simulink model "A21_S7905713_S8999827"  (R2025b)
settings: Solver=VariableStepAuto  StartTime=0.0  StopTime=10.0  RelTol=1e-3
undefined symbols (not defined in the file): X, Y, Z
libraries: nesl_utility x31, sm_lib x27, robotcorelib x1, simulink x1
settings Model: Creator=lucaa  LastModifiedBy=lucaa

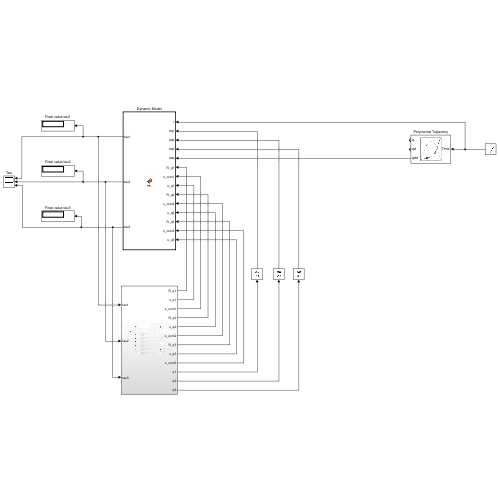
[thumbnail: Simulink's stored preview of the top-level diagram]
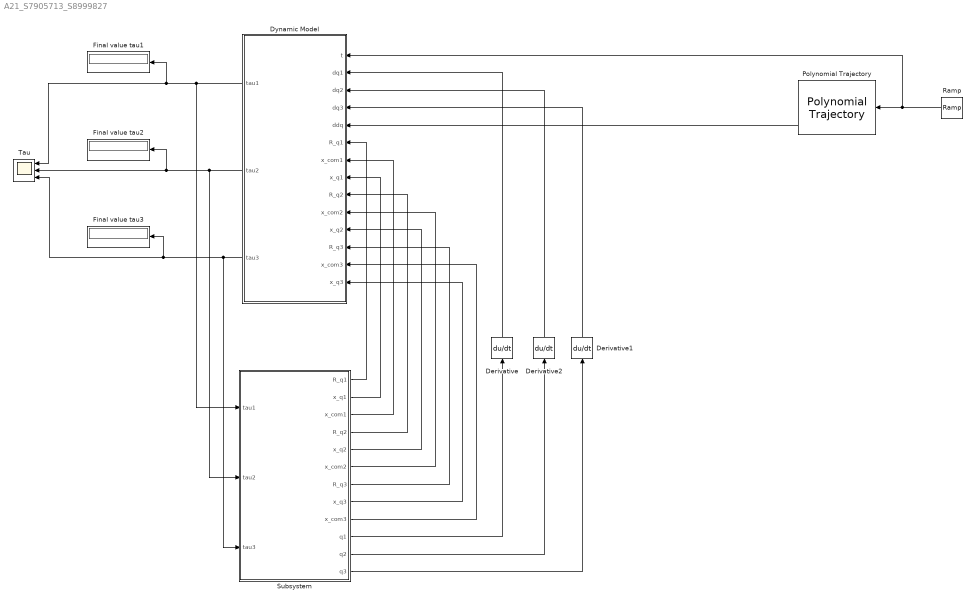
== system A21_S7905713_S8999827 ==
  Derivative : Derivative
  Derivative1 : Derivative
  Derivative2 : Derivative
  Dynamic Model : MATLAB Function  TreatAsAtomicUnit=on
  Final value tau1 : Display
  Final value tau2 : Display
  Final value tau3 : Display
  Polynomial Trajectory : robotcorelib/Polynomial Trajectory  WaypointSource=Internal  Waypoints=[pi/9,pi/3;pi/6,-(pi/180)*15;-(pi/18),(pi/9)*2]  TimePoints=[0,10]  TimeInterval=[ 1, 4 ]  Method=Cubic Polynomial  ParameterSource=Internal  VelocityBoundaryCondition=zeros( 3,2 )  AccelerationBoundaryCondition=zeros( 2, 5 )  SimulateUsing=Interpreted execution
  Ramp : simulink/Sources/Ramp  slope=1  start=0  InitialOutput=0
  Subsystem : Subsystem
  Tau : Scope  NumInputPorts=3
      settings: ActiveDisplayYMinimum=-52.940728526293412  ActiveDisplayYMaximum=68.833359173627684
  wires:
  Subsystem/6(x_com2) -> Dynamic Model/10(x_com2)
  Subsystem/1(R_q1) -> Dynamic Model/6(R_q1)
  Subsystem/4(R_q2) -> Dynamic Model/9(R_q2)
  Subsystem/3(x_com1) -> Dynamic Model/7(x_com1)
  Subsystem/5(x_q2) -> Dynamic Model/11(x_q2)
  Dynamic Model/1(tau1) -> Tau/1, Final value tau1/1, Subsystem/1(tau1)
  Subsystem/2(x_q1) -> Dynamic Model/8(x_q1)
  Dynamic Model/2(tau2) -> Tau/2, Final value tau2/1, Subsystem/2(tau2)
  Polynomial Trajectory/3 -> Dynamic Model/5(ddq)
  Subsystem/7(R_q3) -> Dynamic Model/12(R_q3)
  Subsystem/8(x_q3) -> Dynamic Model/14(x_q3)
  Subsystem/9(x_com3) -> Dynamic Model/13(x_com3)
  Dynamic Model/3(tau3) -> Final value tau3/1, Tau/3, Subsystem/3(tau3)
  Ramp/1 -> Polynomial Trajectory/1, Dynamic Model/1(t)
  Subsystem/10(q1) -> Derivative/1
  Derivative/1 -> Dynamic Model/2(dq1)
  Subsystem/11(q2) -> Derivative2/1
  Subsystem/12(q3) -> Derivative1/1
  Derivative2/1 -> Dynamic Model/3(dq2)
  Derivative1/1 -> Dynamic Model/4(dq3)

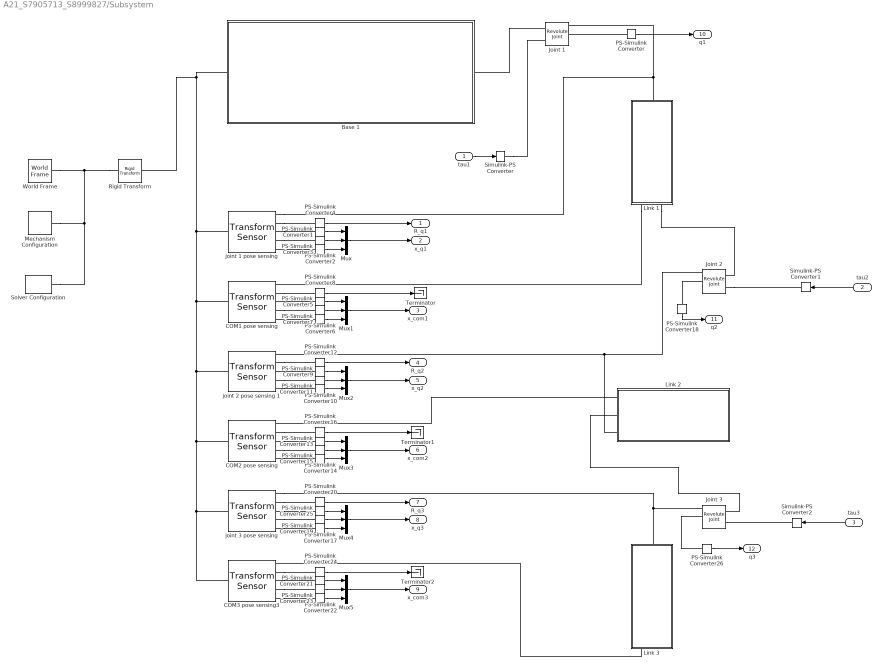
== system A21_S7905713_S8999827/Subsystem ==
  tau1 : Inport
  tau2 : Inport  Port=2
  tau3 : Inport  Port=3
  " Joint 1" : sm_lib/Joints/Revolute Joint  JointMode=Normal  CompositeWrenchDir=FollowerOnBase  CompositeWrenchFrame=BaseFrame  SenseConstraintForce=off  SenseConstraintTorque=off  SenseTotalForce=off  SenseTotalTorque=off  PositionTargetSpecify=on  PositionTargetPriority=High  PositionTargetValue=20  PositionTargetValueUnits=deg  VelocityTargetSpecify=off  VelocityTargetPriority=High  VelocityTargetValue=0  VelocityTargetValueUnits=deg/s  EquilibriumPosition=0  EquilibriumPositionUnits=deg  SpringStiffness=0  SpringStiffnessUnits=N*m/deg  DampingCoefficient=0  DampingCoefficientUnits=N*m/(deg/s)  LowerLimitSpecify=off  LowerLimitBound=-90  LowerLimitBoundUnits=deg  LowerLimitStiffness=1e4  LowerLimitStiffnessUnits=N*m/deg  LowerLimitDamping=10  LowerLimitDampingUnits=N*m/(deg/s)  LowerLimitTransitionRegionWidth=0.1  LowerLimitTransitionRegionWidthUnits=deg  UpperLimitSpecify=off  UpperLimitBound=90  UpperLimitBoundUnits=deg  UpperLimitStiffness=1e4  UpperLimitStiffnessUnits=N*m/deg  UpperLimitDamping=10  UpperLimitDampingUnits=N*m/(deg/s)  UpperLimitTransitionRegionWidth=0.1  UpperLimitTransitionRegionWidthUnits=deg  TorqueActuationMode=InputTorque  MotionActuationMode=ComputedMotion  SensePosition=on  SenseVelocity=off  SenseAcceleration=off  SenseTorqueForce=on  SenseLowerLimitTorqueForce=off  SenseUpperLimitTorqueForce=off
  " Joint 2" : sm_lib/Joints/Revolute Joint  JointMode=Normal  CompositeWrenchDir=FollowerOnBase  CompositeWrenchFrame=BaseFrame  SenseConstraintForce=off  SenseConstraintTorque=off  SenseTotalForce=off  SenseTotalTorque=off  PositionTargetSpecify=on  PositionTargetPriority=High  PositionTargetValue=30  PositionTargetValueUnits=deg  VelocityTargetSpecify=off  VelocityTargetPriority=High  VelocityTargetValue=0  VelocityTargetValueUnits=deg/s  EquilibriumPosition=0  EquilibriumPositionUnits=deg  SpringStiffness=0  SpringStiffnessUnits=N*m/deg  DampingCoefficient=0  DampingCoefficientUnits=N*m/(deg/s)  LowerLimitSpecify=off  LowerLimitBound=-90  LowerLimitBoundUnits=deg  LowerLimitStiffness=1e4  LowerLimitStiffnessUnits=N*m/deg  LowerLimitDamping=10  LowerLimitDampingUnits=N*m/(deg/s)  LowerLimitTransitionRegionWidth=0.1  LowerLimitTransitionRegionWidthUnits=deg  UpperLimitSpecify=off  UpperLimitBound=90  UpperLimitBoundUnits=deg  UpperLimitStiffness=1e4  UpperLimitStiffnessUnits=N*m/deg  UpperLimitDamping=10  UpperLimitDampingUnits=N*m/(deg/s)  UpperLimitTransitionRegionWidth=0.1  UpperLimitTransitionRegionWidthUnits=deg  TorqueActuationMode=InputTorque  MotionActuationMode=ComputedMotion  SensePosition=on  SenseVelocity=off  SenseAcceleration=off  SenseTorqueForce=on  SenseLowerLimitTorqueForce=off  SenseUpperLimitTorqueForce=off
  " Joint 3" : sm_lib/Joints/Revolute Joint  JointMode=Normal  CompositeWrenchDir=FollowerOnBase  CompositeWrenchFrame=BaseFrame  SenseConstraintForce=off  SenseConstraintTorque=off  SenseTotalForce=off  SenseTotalTorque=off  PositionTargetSpecify=on  PositionTargetPriority=High  PositionTargetValue=-10  PositionTargetValueUnits=deg  VelocityTargetSpecify=off  VelocityTargetPriority=High  VelocityTargetValue=0  VelocityTargetValueUnits=deg/s  EquilibriumPosition=0  EquilibriumPositionUnits=deg  SpringStiffness=0  SpringStiffnessUnits=N*m/deg  DampingCoefficient=0  DampingCoefficientUnits=N*m/(deg/s)  LowerLimitSpecify=off  LowerLimitBound=-90  LowerLimitBoundUnits=deg  LowerLimitStiffness=1e4  LowerLimitStiffnessUnits=N*m/deg  LowerLimitDamping=10  LowerLimitDampingUnits=N*m/(deg/s)  LowerLimitTransitionRegionWidth=0.1  LowerLimitTransitionRegionWidthUnits=deg  UpperLimitSpecify=off  UpperLimitBound=90  UpperLimitBoundUnits=deg  UpperLimitStiffness=1e4  UpperLimitStiffnessUnits=N*m/deg  UpperLimitDamping=10  UpperLimitDampingUnits=N*m/(deg/s)  UpperLimitTransitionRegionWidth=0.1  UpperLimitTransitionRegionWidthUnits=deg  TorqueActuationMode=InputTorque  MotionActuationMode=ComputedMotion  SensePosition=on  SenseVelocity=off  SenseAcceleration=off  SenseTorqueForce=on  SenseLowerLimitTorqueForce=off  SenseUpperLimitTorqueForce=off
  Base 1 : Subsystem
  COM1 pose sensing : sm_lib/Frames and Transforms/Transform Sensor  MeasurementFrame=Base  RotationSequence=XYX  SenseAngle=off  SenseAxis=off  SenseQ=off  SenseR=on  SenseRotationSequence=off  SenseOmegaX=off  SenseOmegaY=off  SenseOmegaZ=off  SenseOmega=off  SenseQDot=off  SenseRDot=off  SenseRotationSequenceDot=off  SenseAlphaX=off  SenseAlphaY=off  SenseAlphaZ=off  SenseAlpha=off  SenseQDDot=off  SenseRDDot=off  SenseX=on  SenseY=on  SenseZ=on  SenseXYZ=off  SenseRad=off  SenseAzim=off  SenseDist=off  SenseInc=off  SenseXDot=off  SenseYDot=off  SenseZDot=off  SenseXYZDot=off  SenseRadDot=off  SenseAzimDot=off  SenseDistDot=off  SenseIncDot=off  SenseXDDot=off  SenseYDDot=off  SenseZDDot=off  SenseXYZDDot=off  SenseRadDDot=off  SenseAzimDDot=off  SenseDistDDot=off  SenseIncDDot=off
  COM2 pose sensing : sm_lib/Frames and Transforms/Transform Sensor  MeasurementFrame=Base  RotationSequence=XYX  SenseAngle=off  SenseAxis=off  SenseQ=off  SenseR=on  SenseRotationSequence=off  SenseOmegaX=off  SenseOmegaY=off  SenseOmegaZ=off  SenseOmega=off  SenseQDot=off  SenseRDot=off  SenseRotationSequenceDot=off  SenseAlphaX=off  SenseAlphaY=off  SenseAlphaZ=off  SenseAlpha=off  SenseQDDot=off  SenseRDDot=off  SenseX=on  SenseY=on  SenseZ=on  SenseXYZ=off  SenseRad=off  SenseAzim=off  SenseDist=off  SenseInc=off  SenseXDot=off  SenseYDot=off  SenseZDot=off  SenseXYZDot=off  SenseRadDot=off  SenseAzimDot=off  SenseDistDot=off  SenseIncDot=off  SenseXDDot=off  SenseYDDot=off  SenseZDDot=off  SenseXYZDDot=off  SenseRadDDot=off  SenseAzimDDot=off  SenseDistDDot=off  SenseIncDDot=off
  COM3 pose sensing3 : sm_lib/Frames and Transforms/Transform Sensor  MeasurementFrame=Base  RotationSequence=XYX  SenseAngle=off  SenseAxis=off  SenseQ=off  SenseR=on  SenseRotationSequence=off  SenseOmegaX=off  SenseOmegaY=off  SenseOmegaZ=off  SenseOmega=off  SenseQDot=off  SenseRDot=off  SenseRotationSequenceDot=off  SenseAlphaX=off  SenseAlphaY=off  SenseAlphaZ=off  SenseAlpha=off  SenseQDDot=off  SenseRDDot=off  SenseX=on  SenseY=on  SenseZ=on  SenseXYZ=off  SenseRad=off  SenseAzim=off  SenseDist=off  SenseInc=off  SenseXDot=off  SenseYDot=off  SenseZDot=off  SenseXYZDot=off  SenseRadDot=off  SenseAzimDot=off  SenseDistDot=off  SenseIncDot=off  SenseXDDot=off  SenseYDDot=off  SenseZDDot=off  SenseXYZDDot=off  SenseRadDDot=off  SenseAzimDDot=off  SenseDistDDot=off  SenseIncDDot=off
  Link 1 : Subsystem
  Link 2 : Subsystem
  Link 3 : Subsystem
  Mechanism Configuration : sm_lib/Utilities/Mechanism Configuration  UniformGravity=Constant  GravityVector=[0 0 -9.80665]  GravityVectorUnits=m/s^2  LinearizationDelta=0.001  JointModeTransitionNonlinearIterations=2
  Mux{,1..5} (6 alike) : Mux  Inputs=3
  PS-Simulink Converter{,1..26} (27 alike) : nesl_utility/PS-Simulink Converter  PhysicalDomain=network_engine_domain  SubClassName=ps_output  LeftPortType=input  RightPortType=output  PseudoPeriodic=off  Frequencies=[]  VectorFormat=inherit  Unit=inherit  AffineConversion=off
  Rigid Transform : sm_lib/Frames and Transforms/Rigid Transform  RotationMethod=AlignedAxes  FollAlignAxisA=+Z  BaseAlignAxisA=-Y  FollAlignAxisB=+X  BaseAlignAxisB=+X  RotationStandardAxis=+Z  RotationAngle=0  RotationAngleUnits=deg  RotationArbitraryAxis=[0 0 1]  RotationSequenceAxes=FollowerAxes  RotationSequence=XYX  RotationSequenceAngles=[0 0 0]  RotationSequenceAnglesUnits=deg  RotationMatrix=[1 0 0;0 1 0;0 0 1]  Quaternion=[1 0 0 0]  TranslationMethod=None  TranslationCartesianOffset=[0 0 0]  TranslationCartesianOffsetUnits=m  TranslationStandardAxis=+Z  TranslationStandardOffset=0  TranslationStandardOffsetUnits=m  TranslationROffset=0  TranslationROffsetUnits=m  TranslationThetaOffset=0  TranslationThetaOffsetUnits=deg  TranslationZOffset=0  TranslationZOffsetUnits=m
  Simulink-PS Converter : nesl_utility/Simulink-PS Converter  PhysicalDomain=network_engine_domain  SubClassName=ps_input  LeftPortType=input  RightPortType=output  PseudoPeriodic=off  Frequencies=[]  NoiseDistribution=none  NoiseParameters=[]  Unit=1  AffineConversion=off  FilteringAndDerivatives=provide  SimscapeFilterOrder=1  InputFilterTimeConstant=0.001  UdotUserProvided=0
  Simulink-PS Converter1 : nesl_utility/Simulink-PS Converter  PhysicalDomain=network_engine_domain  SubClassName=ps_input  LeftPortType=input  RightPortType=output  PseudoPeriodic=off  Frequencies=[]  NoiseDistribution=none  NoiseParameters=[]  Unit=1  AffineConversion=off  FilteringAndDerivatives=provide  SimscapeFilterOrder=1  InputFilterTimeConstant=0.001  UdotUserProvided=0
  Simulink-PS Converter2 : nesl_utility/Simulink-PS Converter  PhysicalDomain=network_engine_domain  SubClassName=ps_input  LeftPortType=input  RightPortType=output  PseudoPeriodic=off  Frequencies=[]  NoiseDistribution=none  NoiseParameters=[]  Unit=1  AffineConversion=off  FilteringAndDerivatives=provide  SimscapeFilterOrder=1  InputFilterTimeConstant=0.001  UdotUserProvided=0
  Solver Configuration : nesl_utility/Solver Configuration  PhysicalDomain=network_engine_domain  SubClassName=solver  LeftPortType=input  RightPortType=generic  Tones=[]  Harmonics=[]  SimulateNoise=off  Profile=off  UseLocalSampling=off  EnableSwitchedLinearOptims=on  FrequencyDomain=off  UseCCode=off  RelTol=0.001  AbsTol=0.001  MinStep=1e-09  ToWorkspace=off  RevertToSquareIcSolve=off  NumHomotopyIterations=100  PhasorMode=off  PhasorModeNumHarmonics=1  ConsistencySolver=NEWTON_XTOL_AFTER_FTOL  IndexReductionMethod=DerivativeReplacement  DoDC=off  ResidualTolerance=1e-09  ConsistencyTolSource=GLOBAL  ConsistencyAbsTol=0.001  ConsistencyRelTol=0.001  ConsistencyTolFactor=0.001  UseLocalSolver=off  LocalSolverChoice=NE_BACKWARD_EULER_ADVANCER  ResolveIndetEquations=on  FunctionEvalNumThread=1  LocalSolverSampleTime=0.001  DoFixedCost=off  MaxNonlinIter=3  MaxModeIter=2  ComputeImpulses=off  ImpulseIterations=2  LinearAlgebra=auto  LinearAlgebraNumThread=0  EquationFormulation=NE_TIME_EF  DelaysMemoryBudget=1024  AutomaticFiltering=on  FilteringTimeConstant=0.001  PartitionStorageMethod=AS_NEEDED  PartitionMemoryBudget=1024  PartitionMethod=ROBUST  MultibodyUseLocalSolver=off  MultibodyLocalSolverChoice=ODE1  MultibodyLocalSolverSampleTime=0.001
  Terminator : Terminator
  Terminator1 : Terminator
  Terminator2 : Terminator
  World Frame : sm_lib/Frames and Transforms/World Frame
  "joint 1 pose sensing " : sm_lib/Frames and Transforms/Transform Sensor  MeasurementFrame=Base  RotationSequence=XYX  SenseAngle=off  SenseAxis=off  SenseQ=off  SenseR=on  SenseRotationSequence=off  SenseOmegaX=off  SenseOmegaY=off  SenseOmegaZ=off  SenseOmega=off  SenseQDot=off  SenseRDot=off  SenseRotationSequenceDot=off  SenseAlphaX=off  SenseAlphaY=off  SenseAlphaZ=off  SenseAlpha=off  SenseQDDot=off  SenseRDDot=off  SenseX=on  SenseY=on  SenseZ=on  SenseXYZ=off  SenseRad=off  SenseAzim=off  SenseDist=off  SenseInc=off  SenseXDot=off  SenseYDot=off  SenseZDot=off  SenseXYZDot=off  SenseRadDot=off  SenseAzimDot=off  SenseDistDot=off  SenseIncDot=off  SenseXDDot=off  SenseYDDot=off  SenseZDDot=off  SenseXYZDDot=off  SenseRadDDot=off  SenseAzimDDot=off  SenseDistDDot=off  SenseIncDDot=off
  joint 2 pose sensing 1 : sm_lib/Frames and Transforms/Transform Sensor  MeasurementFrame=Base  RotationSequence=XYX  SenseAngle=off  SenseAxis=off  SenseQ=off  SenseR=on  SenseRotationSequence=off  SenseOmegaX=off  SenseOmegaY=off  SenseOmegaZ=off  SenseOmega=off  SenseQDot=off  SenseRDot=off  SenseRotationSequenceDot=off  SenseAlphaX=off  SenseAlphaY=off  SenseAlphaZ=off  SenseAlpha=off  SenseQDDot=off  SenseRDDot=off  SenseX=on  SenseY=on  SenseZ=on  SenseXYZ=off  SenseRad=off  SenseAzim=off  SenseDist=off  SenseInc=off  SenseXDot=off  SenseYDot=off  SenseZDot=off  SenseXYZDot=off  SenseRadDot=off  SenseAzimDot=off  SenseDistDot=off  SenseIncDot=off  SenseXDDot=off  SenseYDDot=off  SenseZDDot=off  SenseXYZDDot=off  SenseRadDDot=off  SenseAzimDDot=off  SenseDistDDot=off  SenseIncDDot=off
  joint 3 pose sensing : sm_lib/Frames and Transforms/Transform Sensor  MeasurementFrame=Base  RotationSequence=XYX  SenseAngle=off  SenseAxis=off  SenseQ=off  SenseR=on  SenseRotationSequence=off  SenseOmegaX=off  SenseOmegaY=off  SenseOmegaZ=off  SenseOmega=off  SenseQDot=off  SenseRDot=off  SenseRotationSequenceDot=off  SenseAlphaX=off  SenseAlphaY=off  SenseAlphaZ=off  SenseAlpha=off  SenseQDDot=off  SenseRDDot=off  SenseX=on  SenseY=on  SenseZ=on  SenseXYZ=off  SenseRad=off  SenseAzim=off  SenseDist=off  SenseInc=off  SenseXDot=off  SenseYDot=off  SenseZDot=off  SenseXYZDot=off  SenseRadDot=off  SenseAzimDot=off  SenseDistDot=off  SenseIncDot=off  SenseXDDot=off  SenseYDDot=off  SenseZDDot=off  SenseXYZDDot=off  SenseRadDDot=off  SenseAzimDDot=off  SenseDistDDot=off  SenseIncDDot=off
  R_q1 : Outport
  x_q1 : Outport  Port=2
  x_com1 : Outport  Port=3
  R_q2 : Outport  Port=4
  x_q2 : Outport  Port=5
  x_com2 : Outport  Port=6
  R_q3 : Outport  Port=7
  x_q3 : Outport  Port=8
  x_com3 : Outport  Port=9
  q1 : Outport  Port=10
  q2 : Outport  Port=11
  q3 : Outport  Port=12
  wires:
  PS-Simulink Converter2/1 -> Mux/2
  PS-Simulink Converter6/1 -> Mux1/2
  PS-Simulink Converter7/1 -> Mux1/3
  PS-Simulink Converter8/1 -> Terminator/1
  Mux/1 -> x_q1/1
  PS-Simulink Converter4/1 -> R_q1/1
  PS-Simulink Converter1/1 -> Mux/1
  PS-Simulink Converter5/1 -> Mux1/1
  Mux1/1 -> x_com1/1
  PS-Simulink Converter3/1 -> Mux/3
  tau1/1 -> Simulink-PS Converter/1
  PS-Simulink Converter11/1 -> Mux2/3
  PS-Simulink Converter16/1 -> Terminator1/1
  PS-Simulink Converter10/1 -> Mux2/2
  Mux3/1 -> x_com2/1
  PS-Simulink Converter13/1 -> Mux3/1
  tau2/1 -> Simulink-PS Converter1/1
  PS-Simulink Converter9/1 -> Mux2/1
  PS-Simulink Converter12/1 -> R_q2/1
  Mux2/1 -> x_q2/1
  PS-Simulink Converter15/1 -> Mux3/3
  PS-Simulink Converter14/1 -> Mux3/2
  PS-Simulink Converter22/1 -> Mux5/2
  Mux5/1 -> x_com3/1
  PS-Simulink Converter25/1 -> Mux4/1
  Mux4/1 -> x_q3/1
  PS-Simulink Converter19/1 -> Mux4/3
  PS-Simulink Converter17/1 -> Mux4/2
  PS-Simulink Converter21/1 -> Mux5/1
  PS-Simulink Converter24/1 -> Terminator2/1
  PS-Simulink Converter20/1 -> R_q3/1
  PS-Simulink Converter23/1 -> Mux5/3
  tau3/1 -> Simulink-PS Converter2/1
  PS-Simulink Converter/1 -> q1/1
  PS-Simulink Converter18/1 -> q2/1
  PS-Simulink Converter26/1 -> q3/1
  connections:
  Rigid Transform/LConn1 -- World Frame/RConn1 -- Solver Configuration/RConn1 -- Mechanism Configuration/RConn1
  "joint 1 pose sensing "/RConn5 -- PS-Simulink Converter3/LConn1
  COM1 pose sensing/RConn3 -- PS-Simulink Converter5/LConn1
  COM1 pose sensing/RConn2 -- PS-Simulink Converter8/LConn1
  "joint 1 pose sensing "/RConn2 -- PS-Simulink Converter4/LConn1
  COM1 pose sensing/RConn5 -- PS-Simulink Converter7/LConn1
  Simulink-PS Converter/RConn1 -- " Joint 1"/LConn2
  " Joint 1"/LConn1 -- Base 1/RConn1
  Link 1/RConn1 -- COM1 pose sensing/RConn1
  COM1 pose sensing/RConn4 -- PS-Simulink Converter6/LConn1
  "joint 1 pose sensing "/RConn3 -- PS-Simulink Converter1/LConn1
  "joint 1 pose sensing "/RConn4 -- PS-Simulink Converter2/LConn1
  Link 2/RConn3 -- " Joint 2"/RConn1 -- joint 2 pose sensing 1/RConn1
  COM2 pose sensing/RConn3 -- PS-Simulink Converter13/LConn1
  joint 2 pose sensing 1/RConn4 -- PS-Simulink Converter10/LConn1
  Link 2/RConn1 -- COM2 pose sensing/RConn1
  joint 2 pose sensing 1/RConn2 -- PS-Simulink Converter12/LConn1
  joint 2 pose sensing 1/RConn5 -- PS-Simulink Converter11/LConn1
  COM2 pose sensing/RConn5 -- PS-Simulink Converter15/LConn1
  COM2 pose sensing/RConn4 -- PS-Simulink Converter14/LConn1
  COM2 pose sensing/RConn2 -- PS-Simulink Converter16/LConn1
  joint 2 pose sensing 1/RConn3 -- PS-Simulink Converter9/LConn1
  " Joint 2"/LConn2 -- Simulink-PS Converter1/RConn1
  Link 1/RConn2 -- " Joint 2"/LConn1
  Link 1/LConn1 -- " Joint 1"/RConn1 -- "joint 1 pose sensing "/RConn1
  "joint 1 pose sensing "/LConn1 -- COM1 pose sensing/LConn1 -- COM3 pose sensing3/LConn1 -- joint 3 pose sensing/LConn1 -- COM2 pose sensing/LConn1 -- joint 2 pose sensing 1/LConn1 -- Base 1/LConn1 -- Rigid Transform/RConn1
  joint 3 pose sensing/RConn2 -- PS-Simulink Converter20/LConn1
  joint 3 pose sensing/RConn3 -- PS-Simulink Converter25/LConn1
  joint 3 pose sensing/RConn5 -- PS-Simulink Converter19/LConn1
  joint 3 pose sensing/RConn4 -- PS-Simulink Converter17/LConn1
  COM3 pose sensing3/RConn2 -- PS-Simulink Converter24/LConn1
  COM3 pose sensing3/RConn5 -- PS-Simulink Converter23/LConn1
  COM3 pose sensing3/RConn3 -- PS-Simulink Converter21/LConn1
  COM3 pose sensing3/RConn4 -- PS-Simulink Converter22/LConn1
  Link 2/RConn2 -- " Joint 3"/LConn1
  Simulink-PS Converter2/RConn1 -- " Joint 3"/LConn2
  " Joint 3"/RConn1 -- Link 3/LConn1 -- joint 3 pose sensing/RConn1
  Link 3/RConn1 -- COM3 pose sensing3/RConn1
  PS-Simulink Converter/LConn1 -- " Joint 1"/RConn2
  " Joint 2"/RConn2 -- PS-Simulink Converter18/LConn1
  " Joint 3"/RConn2 -- PS-Simulink Converter26/LConn1

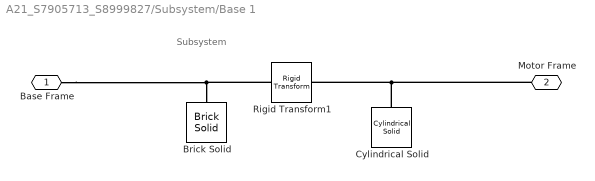
== system A21_S7905713_S8999827/Subsystem/Base 1 ==
  note: Subsystem
  Brick Solid : sm_lib/Body Elements/Brick Solid  BrickDimensions=[50 50 10]  BrickDimensionsUnits=cm  ExportEntireGeometry=off  InertiaType=PointMass  BasedOnType=Mass  Density=1000  DensityUnits=kg/m^3  Mass=0  MassUnits=kg  CenterOfMass=[0 0 0]  CenterOfMassUnits=m  MomentsOfInertia=[1 1 1]  MomentsOfInertiaUnits=kg*m^2  ProductsOfInertia=[0 0 0]  ProductsOfInertiaUnits=kg*m^2  GraphicType=FromGeometry  MarkerShape=Sphere  MarkerSize=10  GraphicVisPropType=SimpleVisualProperties  GraphicDiffuseColor=[0.6667 0.4745 0.2588]  GraphicOpacity=1  GraphicSpecularColor=[0.5 0.5 0.5 1.0]  GraphicAmbientColor=[0.15 0.15 0.15 1.0]  GraphicEmissiveColor=[0.0 0.0 0.0 1.0]  GraphicShininess=75  DoExposeReferenceFrame=on  SerializedFrames=<Frames/>
  Cylindrical Solid : sm_lib/Body Elements/Cylindrical Solid  CylinderRadius=5  CylinderRadiusUnits=cm  CylinderLength=10  CylinderLengthUnits=cm  ExportEntireGeometry=off  InertiaType=PointMass  BasedOnType=Mass  Density=1000  DensityUnits=kg/m^3  Mass=0  MassUnits=kg  CenterOfMass=[0 0 0]  CenterOfMassUnits=m  MomentsOfInertia=[1 1 1]  MomentsOfInertiaUnits=kg*m^2  ProductsOfInertia=[0 0 0]  ProductsOfInertiaUnits=kg*m^2  GraphicType=FromGeometry  MarkerShape=Sphere  MarkerSize=10  GraphicVisPropType=SimpleVisualProperties  GraphicDiffuseColor=[0.01569 0.2 1]  GraphicOpacity=1  GraphicSpecularColor=[0.5 0.5 0.5 1.0]  GraphicAmbientColor=[0.15 0.15 0.15 1.0]  GraphicEmissiveColor=[0.0 0.0 0.0 1.0]  GraphicShininess=75  DoExposeReferenceFrame=on  SerializedFrames=<Frames/>
  Rigid Transform1 : sm_lib/Frames and Transforms/Rigid Transform  RotationMethod=None  FollAlignAxisA=+Z  BaseAlignAxisA=+X  FollAlignAxisB=+Y  BaseAlignAxisB=+Y  RotationStandardAxis=+Z  RotationAngle=0  RotationAngleUnits=deg  RotationArbitraryAxis=[0 0 1]  RotationSequenceAxes=FollowerAxes  RotationSequence=XYX  RotationSequenceAngles=[0 0 0]  RotationSequenceAnglesUnits=deg  RotationMatrix=[1 0 0;0 1 0;0 0 1]  Quaternion=[1 0 0 0]  TranslationMethod=Cartesian  TranslationCartesianOffset=[0 0 7.5]  TranslationCartesianOffsetUnits=cm  TranslationStandardAxis=+Z  TranslationStandardOffset=0  TranslationStandardOffsetUnits=m  TranslationROffset=0  TranslationROffsetUnits=m  TranslationThetaOffset=0  TranslationThetaOffsetUnits=deg  TranslationZOffset=0  TranslationZOffsetUnits=m
  Base Frame : PMIOPort  Side=Left
  " Motor Frame" : PMIOPort  Port=2  Side=Right
  connections:
  Rigid Transform1/LConn1 -- Base Frame/RConn1 -- Brick Solid/RConn1
  Cylindrical Solid/RConn1 -- " Motor Frame"/RConn1 -- Rigid Transform1/RConn1

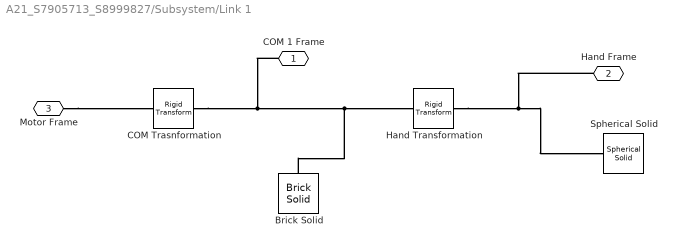
== system A21_S7905713_S8999827/Subsystem/Link 1 ==
  Brick Solid : sm_lib/Body Elements/Brick Solid  BrickDimensions=[20 1 1]  BrickDimensionsUnits=cm  ExportEntireGeometry=off  InertiaType=CalculateFromGeometry  BasedOnType=Mass  Density=1000  DensityUnits=kg/m^3  Mass=2.5  MassUnits=kg  CenterOfMass=[0 0 0]  CenterOfMassUnits=m  MomentsOfInertia=[1 1 1]  MomentsOfInertiaUnits=kg*m^2  ProductsOfInertia=[0 0 0]  ProductsOfInertiaUnits=kg*m^2  GraphicType=FromGeometry  MarkerShape=Sphere  MarkerSize=10  GraphicVisPropType=SimpleVisualProperties  GraphicDiffuseColor=[1 0.149 0]  GraphicOpacity=1  GraphicSpecularColor=[0.5 0.5 0.5 1.0]  GraphicAmbientColor=[0.15 0.15 0.15 1.0]  GraphicEmissiveColor=[0.0 0.0 0.0 1.0]  GraphicShininess=75  DoExposeReferenceFrame=on  SerializedFrames=<Frames/>
  COM Trasnformation : sm_lib/Frames and Transforms/Rigid Transform  RotationMethod=None  FollAlignAxisA=+Z  BaseAlignAxisA=-Y  FollAlignAxisB=+X  BaseAlignAxisB=+X  RotationStandardAxis=+Z  RotationAngle=0  RotationAngleUnits=deg  RotationArbitraryAxis=[0 0 1]  RotationSequenceAxes=FollowerAxes  RotationSequence=XYX  RotationSequenceAngles=[0 0 0]  RotationSequenceAnglesUnits=deg  RotationMatrix=[1 0 0;0 1 0;0 0 1]  Quaternion=[1 0 0 0]  TranslationMethod=Cartesian  TranslationCartesianOffset=[10 0 0]  TranslationCartesianOffsetUnits=cm  TranslationStandardAxis=+Z  TranslationStandardOffset=0  TranslationStandardOffsetUnits=m  TranslationROffset=0  TranslationROffsetUnits=m  TranslationThetaOffset=0  TranslationThetaOffsetUnits=deg  TranslationZOffset=0  TranslationZOffsetUnits=m
  Hand Transformation : sm_lib/Frames and Transforms/Rigid Transform  RotationMethod=None  FollAlignAxisA=+Z  BaseAlignAxisA=-Y  FollAlignAxisB=+X  BaseAlignAxisB=+X  RotationStandardAxis=+Z  RotationAngle=0  RotationAngleUnits=deg  RotationArbitraryAxis=[0 0 1]  RotationSequenceAxes=FollowerAxes  RotationSequence=XYX  RotationSequenceAngles=[0 0 0]  RotationSequenceAnglesUnits=deg  RotationMatrix=[1 0 0;0 1 0;0 0 1]  Quaternion=[1 0 0 0]  TranslationMethod=Cartesian  TranslationCartesianOffset=[10 0 0]  TranslationCartesianOffsetUnits=cm  TranslationStandardAxis=+Z  TranslationStandardOffset=0  TranslationStandardOffsetUnits=m  TranslationROffset=0  TranslationROffsetUnits=m  TranslationThetaOffset=0  TranslationThetaOffsetUnits=deg  TranslationZOffset=0  TranslationZOffsetUnits=m
  Spherical Solid : sm_lib/Body Elements/Spherical Solid  SphereRadius=2  SphereRadiusUnits=cm  ExportEntireGeometry=off  InertiaType=CalculateFromGeometry  BasedOnType=Mass  Density=1000  DensityUnits=kg/m^3  Mass=0  MassUnits=kg  CenterOfMass=[0 0 0]  CenterOfMassUnits=m  MomentsOfInertia=[1 1 1]  MomentsOfInertiaUnits=kg*m^2  ProductsOfInertia=[0 0 0]  ProductsOfInertiaUnits=kg*m^2  GraphicType=FromGeometry  MarkerShape=Sphere  MarkerSize=10  GraphicVisPropType=SimpleVisualProperties  GraphicDiffuseColor=[0.01569 0.2 1]  GraphicOpacity=1  GraphicSpecularColor=[0.5 0.5 0.5 1.0]  GraphicAmbientColor=[0.15 0.15 0.15 1.0]  GraphicEmissiveColor=[0.0 0.0 0.0 1.0]  GraphicShininess=75  DoExposeReferenceFrame=on  SerializedFrames=<Frames/>
  COM 1 Frame : PMIOPort  Side=Right
  "Hand Frame " : PMIOPort  Port=2  Side=Right
  Motor Frame : PMIOPort  Port=3  Side=Left
  connections:
  Motor Frame/RConn1 -- COM Trasnformation/LConn1
  Hand Transformation/RConn1 -- "Hand Frame "/RConn1 -- Spherical Solid/RConn1
  COM Trasnformation/RConn1 -- COM 1 Frame/RConn1 -- Brick Solid/RConn1 -- Hand Transformation/LConn1

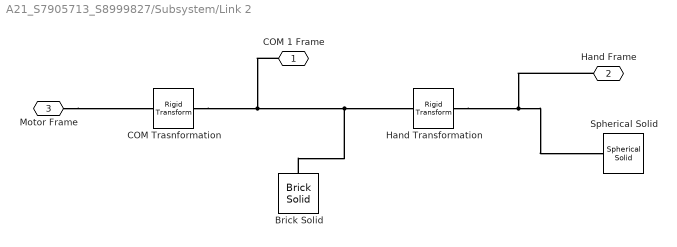
== system A21_S7905713_S8999827/Subsystem/Link 2 ==
  Brick Solid : sm_lib/Body Elements/Brick Solid  BrickDimensions=[20 1 1]  BrickDimensionsUnits=cm  ExportEntireGeometry=off  InertiaType=CalculateFromGeometry  BasedOnType=Mass  Density=1000  DensityUnits=kg/m^3  Mass=4.5  MassUnits=kg  CenterOfMass=[0 0 0]  CenterOfMassUnits=m  MomentsOfInertia=[1 1 1]  MomentsOfInertiaUnits=kg*m^2  ProductsOfInertia=[0 0 0]  ProductsOfInertiaUnits=kg*m^2  GraphicType=FromGeometry  MarkerShape=Sphere  MarkerSize=10  GraphicVisPropType=SimpleVisualProperties  GraphicDiffuseColor=[1 0.149 0]  GraphicOpacity=1  GraphicSpecularColor=[0.5 0.5 0.5 1.0]  GraphicAmbientColor=[0.15 0.15 0.15 1.0]  GraphicEmissiveColor=[0.0 0.0 0.0 1.0]  GraphicShininess=75  DoExposeReferenceFrame=on  SerializedFrames=<Frames/>
  COM Trasnformation : sm_lib/Frames and Transforms/Rigid Transform  RotationMethod=None  FollAlignAxisA=+Z  BaseAlignAxisA=-Y  FollAlignAxisB=+X  BaseAlignAxisB=+X  RotationStandardAxis=+Z  RotationAngle=0  RotationAngleUnits=deg  RotationArbitraryAxis=[0 0 1]  RotationSequenceAxes=FollowerAxes  RotationSequence=XYX  RotationSequenceAngles=[0 0 0]  RotationSequenceAnglesUnits=deg  RotationMatrix=[1 0 0;0 1 0;0 0 1]  Quaternion=[1 0 0 0]  TranslationMethod=Cartesian  TranslationCartesianOffset=[10 0 0]  TranslationCartesianOffsetUnits=cm  TranslationStandardAxis=+Z  TranslationStandardOffset=0  TranslationStandardOffsetUnits=m  TranslationROffset=0  TranslationROffsetUnits=m  TranslationThetaOffset=0  TranslationThetaOffsetUnits=deg  TranslationZOffset=0  TranslationZOffsetUnits=m
  Hand Transformation : sm_lib/Frames and Transforms/Rigid Transform  RotationMethod=None  FollAlignAxisA=+Z  BaseAlignAxisA=-Y  FollAlignAxisB=+X  BaseAlignAxisB=+X  RotationStandardAxis=+Z  RotationAngle=0  RotationAngleUnits=deg  RotationArbitraryAxis=[0 0 1]  RotationSequenceAxes=FollowerAxes  RotationSequence=XYX  RotationSequenceAngles=[0 0 0]  RotationSequenceAnglesUnits=deg  RotationMatrix=[1 0 0;0 1 0;0 0 1]  Quaternion=[1 0 0 0]  TranslationMethod=Cartesian  TranslationCartesianOffset=[10 0 0]  TranslationCartesianOffsetUnits=cm  TranslationStandardAxis=+Z  TranslationStandardOffset=0  TranslationStandardOffsetUnits=m  TranslationROffset=0  TranslationROffsetUnits=m  TranslationThetaOffset=0  TranslationThetaOffsetUnits=deg  TranslationZOffset=0  TranslationZOffsetUnits=m
  Spherical Solid : sm_lib/Body Elements/Spherical Solid  SphereRadius=2  SphereRadiusUnits=cm  ExportEntireGeometry=off  InertiaType=CalculateFromGeometry  BasedOnType=Mass  Density=1000  DensityUnits=kg/m^3  Mass=0  MassUnits=kg  CenterOfMass=[0 0 0]  CenterOfMassUnits=m  MomentsOfInertia=[1 1 1]  MomentsOfInertiaUnits=kg*m^2  ProductsOfInertia=[0 0 0]  ProductsOfInertiaUnits=kg*m^2  GraphicType=FromGeometry  MarkerShape=Sphere  MarkerSize=10  GraphicVisPropType=SimpleVisualProperties  GraphicDiffuseColor=[0.01569 0.2 1]  GraphicOpacity=1  GraphicSpecularColor=[0.5 0.5 0.5 1.0]  GraphicAmbientColor=[0.15 0.15 0.15 1.0]  GraphicEmissiveColor=[0.0 0.0 0.0 1.0]  GraphicShininess=75  DoExposeReferenceFrame=on  SerializedFrames=<Frames/>
  COM 1 Frame : PMIOPort  Side=Right
  "Hand Frame " : PMIOPort  Port=2  Side=Right
  Motor Frame : PMIOPort  Port=3  Side=Right
  connections:
  Motor Frame/RConn1 -- COM Trasnformation/LConn1
  Hand Transformation/RConn1 -- "Hand Frame "/RConn1 -- Spherical Solid/RConn1
  COM Trasnformation/RConn1 -- COM 1 Frame/RConn1 -- Brick Solid/RConn1 -- Hand Transformation/LConn1

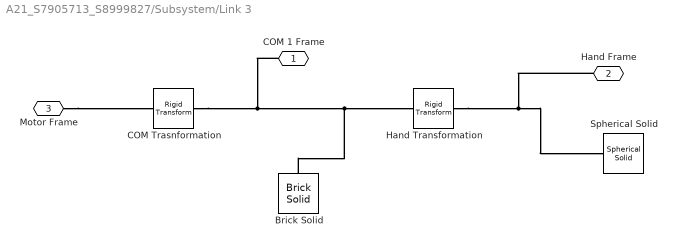
== system A21_S7905713_S8999827/Subsystem/Link 3 ==
  Brick Solid : sm_lib/Body Elements/Brick Solid  BrickDimensions=[20 1 1]  BrickDimensionsUnits=cm  ExportEntireGeometry=off  InertiaType=CalculateFromGeometry  BasedOnType=Mass  Density=1000  DensityUnits=kg/m^3  Mass=1.5  MassUnits=kg  CenterOfMass=[0 0 0]  CenterOfMassUnits=m  MomentsOfInertia=[1 1 1]  MomentsOfInertiaUnits=kg*m^2  ProductsOfInertia=[0 0 0]  ProductsOfInertiaUnits=kg*m^2  GraphicType=FromGeometry  MarkerShape=Sphere  MarkerSize=10  GraphicVisPropType=SimpleVisualProperties  GraphicDiffuseColor=[1 0.149 0]  GraphicOpacity=1  GraphicSpecularColor=[0.5 0.5 0.5 1.0]  GraphicAmbientColor=[0.15 0.15 0.15 1.0]  GraphicEmissiveColor=[0.0 0.0 0.0 1.0]  GraphicShininess=75  DoExposeReferenceFrame=on  SerializedFrames=<Frames/>
  COM Trasnformation : sm_lib/Frames and Transforms/Rigid Transform  RotationMethod=None  FollAlignAxisA=+Z  BaseAlignAxisA=-Y  FollAlignAxisB=+X  BaseAlignAxisB=+X  RotationStandardAxis=+Z  RotationAngle=0  RotationAngleUnits=deg  RotationArbitraryAxis=[0 0 1]  RotationSequenceAxes=FollowerAxes  RotationSequence=XYX  RotationSequenceAngles=[0 0 0]  RotationSequenceAnglesUnits=deg  RotationMatrix=[1 0 0;0 1 0;0 0 1]  Quaternion=[1 0 0 0]  TranslationMethod=Cartesian  TranslationCartesianOffset=[10 0 0]  TranslationCartesianOffsetUnits=cm  TranslationStandardAxis=+Z  TranslationStandardOffset=0  TranslationStandardOffsetUnits=m  TranslationROffset=0  TranslationROffsetUnits=m  TranslationThetaOffset=0  TranslationThetaOffsetUnits=deg  TranslationZOffset=0  TranslationZOffsetUnits=m
  Hand Transformation : sm_lib/Frames and Transforms/Rigid Transform  RotationMethod=None  FollAlignAxisA=+Z  BaseAlignAxisA=-Y  FollAlignAxisB=+X  BaseAlignAxisB=+X  RotationStandardAxis=+Z  RotationAngle=0  RotationAngleUnits=deg  RotationArbitraryAxis=[0 0 1]  RotationSequenceAxes=FollowerAxes  RotationSequence=XYX  RotationSequenceAngles=[0 0 0]  RotationSequenceAnglesUnits=deg  RotationMatrix=[1 0 0;0 1 0;0 0 1]  Quaternion=[1 0 0 0]  TranslationMethod=Cartesian  TranslationCartesianOffset=[10 0 0]  TranslationCartesianOffsetUnits=cm  TranslationStandardAxis=+Z  TranslationStandardOffset=0  TranslationStandardOffsetUnits=m  TranslationROffset=0  TranslationROffsetUnits=m  TranslationThetaOffset=0  TranslationThetaOffsetUnits=deg  TranslationZOffset=0  TranslationZOffsetUnits=m
  Spherical Solid : sm_lib/Body Elements/Spherical Solid  SphereRadius=2  SphereRadiusUnits=cm  ExportEntireGeometry=off  InertiaType=PointMass  BasedOnType=Mass  Density=1000  DensityUnits=kg/m^3  Mass=0  MassUnits=kg  CenterOfMass=[0 0 0]  CenterOfMassUnits=m  MomentsOfInertia=[1 1 1]  MomentsOfInertiaUnits=kg*m^2  ProductsOfInertia=[0 0 0]  ProductsOfInertiaUnits=kg*m^2  GraphicType=FromGeometry  MarkerShape=Sphere  MarkerSize=10  GraphicVisPropType=SimpleVisualProperties  GraphicDiffuseColor=[0.01569 0.2 1]  GraphicOpacity=1  GraphicSpecularColor=[0.5 0.5 0.5 1.0]  GraphicAmbientColor=[0.15 0.15 0.15 1.0]  GraphicEmissiveColor=[0.0 0.0 0.0 1.0]  GraphicShininess=75  DoExposeReferenceFrame=on  SerializedFrames=<Frames/>
  COM 1 Frame : PMIOPort  Side=Right
  "Hand Frame " : PMIOPort  Port=2  Side=Right
  Motor Frame : PMIOPort  Port=3  Side=Left
  connections:
  Motor Frame/RConn1 -- COM Trasnformation/LConn1
  Hand Transformation/RConn1 -- "Hand Frame "/RConn1 -- Spherical Solid/RConn1
  COM Trasnformation/RConn1 -- COM 1 Frame/RConn1 -- Brick Solid/RConn1 -- Hand Transformation/LConn1

== matlab function A21_S7905713_S8999827/Dynamic Model ==
  data: t input; tau1 output; tau2 output; dq1 input; dq2 input; dq3 input; ddq input; R_q1 input; x_com1 input; x_q1 input; R_q2 input; x_com2 input; x_q2 input; R_q3 input; x_com3 input; x_q3 input; tau3 output
%IMPLEMENTATION OF INVVERSE DYNAMIC PORBLEM
function [tau1, tau2, tau3]   = fcn(t, dq1, dq2, dq3, ddq, R_q1, x_com1, x_q1, R_q2, x_com2, x_q2, R_q3, x_com3, x_q3)


%% DATA INITALIZATION

dq=[dq1;dq2;dq3];

m1 = 2.5;
m2 = 4.5;
m3 = 1.5;
m = [m1; m2; m3];    % mass vector

w_0 = [0;0;0];      
dw_0 = [0;0;0];

g = [0;9.80665;0];
n = 3;               %number link

l1 = 0.2;
l2 = 0.2;
l3 = 0.2;
l = [l1; l2; l3];    %link lenght vector

bc_I = zeros(3,3,n); %inertial operator

k = zeros(3,n);      %z-axis

R = zeros(3,3,n+1);      % rotation matrices from i-1 to i
R(:,:,1) = R_q1';        % from 0 to 1
R(:,:,2) = R_q2'*R_q1;   % rotation from 1 to 2 
R(:,:,3) = R_q3'*R_q2;   % from 2 to 3
R(:,:,n+1) = eye(3);     % end effector

for i=1:n
    %inertial operator
    bc_I(:,:,i) = zeros(3);
    %bc_I(2,2, i) = (1/12) * m(i) * l(i)^2;
    bc_I(3,3, i) = (1/12) * m(i) * l(i)^2;

    k(:,i) = [0;0;1];    %z-axis
end

% centers of mass i vectors wrt base i
b_x_com = zeros(3, n);
b_x_com(:,1) = R_q1' *(x_com1 - x_q1);
b_x_com(:,2) = R_q2' *(x_com2 - x_q2);
b_x_com(:,3) = R_q3' *(x_com3 - x_q3);

% r_i_prev_i: vettore che va dal giunto i-1 al giunto i, espresso nel frame i-1
x_rel = zeros(3, n+1);

x_rel(:,1) = [0;0;0.1];     % from base to joint 1
x_rel(:,2) = [0.2;0;0];     % from joint 1 to joint2
x_rel(:,3) = [0.2;0;0];     % from joint 2 to joint 3
x_rel(:,4) = [0;0;0];       % end-effector 

% data for backward and forward computation
w_i_0 = zeros(3,n);
wdot_i_0 = zeros(3,n);
vdot_i_0 = zeros(3,n);
vdot_Ci_0 = zeros(3,n);
F_i = zeros(3,n);
N_i = zeros(3,n);
f = zeros(3, n+1);          %forces of joint i acting on i-1
ni = zeros(3, n+1);         %momentun of joint i acting on i-1

tau = zeros(1,n);

%% FORWARD PROPAGATION

for i=1:n

    if i==1
        w_prev = w_0;
        wdot_prev = dw_0;
        vdot_prev = g; 
    else
        w_prev = w_i_0(:, i-1);
        wdot_prev = wdot_i_0(:, i-1);
        vdot_prev = vdot_i_0(:, i-1);
    end

    w_i_0(:,i) = R(:,:,i)* w_prev + dq(i)*k(:,i);
    % Angolar Acceleration
    wdot_i_0(:,i) = R(:,:,i) * wdot_prev+cross(R(:,:,i)*w_prev, dq(i)*k(:,i))+ ddq(i)* k(:,i);
    % Linear Acceleration
    vdot_i_0(:,i) = R(:,:,i) *(cross(wdot_prev, x_rel(:,i)) + cross(w_prev, cross(w_prev,x_rel(:,i))) + vdot_prev );
    % Linear Acceleration of COM
    vdot_Ci_0(:,i) = cross(wdot_i_0(:,i), b_x_com(:,i)) + cross(w_i_0(:,i), cross(w_i_0(:,i),b_x_com(:,i))) +vdot_i_0(:,i);
    % Force on COM, newton law (intertial force)
    F_i(:,i) = m(i)*vdot_Ci_0(:,i);
    % Torque on COM, newton-euler law (intertial mementum)
    N_i(:,i) = bc_I(:,:,i) * wdot_i_0(:,i) + cross(w_i_0(:,i),bc_I(:,:,i)*w_i_0(:,i));

end

%% BACKWARD PROPAGATION
for i=n:-1:1
    % Force acting on joint i (intertial + force acting on joint i+1)
    f(:,i) = R(:,:,i+1)'*f(:,i+1) + F_i(:,i);
    % Torque action on joint i (inertial + momentum acting on joint i+1 + angular momentum of the inertial     
    ni(:,i) = N_i(:,i) + R(:,:,i+1)'* ni(:,i+1) + cross(b_x_com(:,i), F_i(:,i) ) + cross(x_rel(:,i+1), R(:,:,i+1)'*f(:,i+1)); %ricordarsi di portare tutto rispetto a i
 
    tau(i) = ni(:,i)'*k(:,i);

end


if t==10 
    tau1 = tau(1);
    disp("---------------------");
    disp("tau1 at istant t=10s");
    disp(tau1);
    tau2 = tau(2);
    disp("tau2 at istant t=10s");
    disp(tau2);
    tau3 = tau(3);
    disp("tau3 at istant t=10s");
    disp(tau3);
    disp("---------------------");

end

tau1 = tau(1);
tau2 = tau(2);
tau3 = tau(3);
